simulink model "linsec"  (R2015b)
settings: Solver=VariableStepAuto  StartTime=0.0  StopTime=10.0  RelTol=1e-3
settings Model: Creator=vinayshanbhag  LastModifiedBy=vinayshanbhag

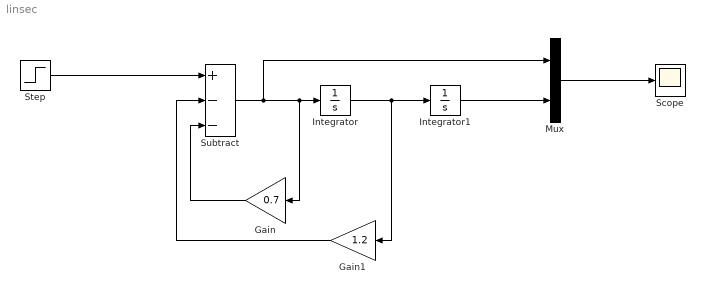
== system linsec ==
  Gain : Gain  Gain=0.7
  "Gain1 " : Gain  Gain=1.2
  Integrator : Integrator
  Integrator1 : Integrator
  Mux : Mux  Inputs=2
  Scope : Scope
  Step : Step  SampleTime=0
  Subtract : Sum  Inputs=+--
  wires:
  Step/1 -> Subtract/1
  Subtract/1 -> Mux/1, Gain/1, Integrator/1
  Integrator/1 -> "Gain1 "/1, Integrator1/1
  Gain/1 -> Subtract/3
  "Gain1 "/1 -> Subtract/2
  Mux/1 -> Scope/1
  Integrator1/1 -> Mux/2
